simulink model "swing_language_control_sim"  (R2025a)
settings: Solver=ode4  StartTime=0.0  StopTime=simDuration  FixedStep=0.1  RelTol=1e-3
values from neighbouring files (symbols this model uses):
  siteMap = jsondecode(fileread(mapPath))    [actionsToVelocityCmd.m]
settings Model: Creator=Lenovo  LastModifiedBy=Lenovo

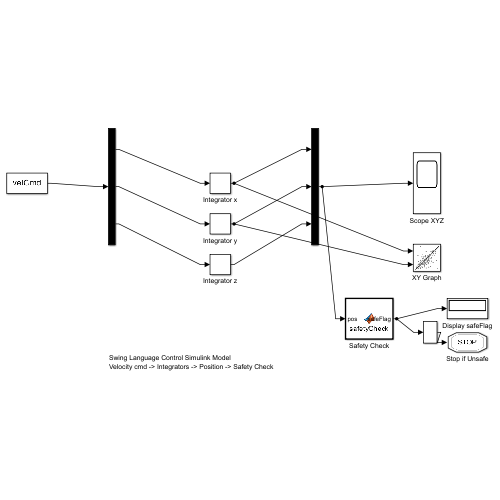
[thumbnail: Simulink's stored preview of the top-level diagram]
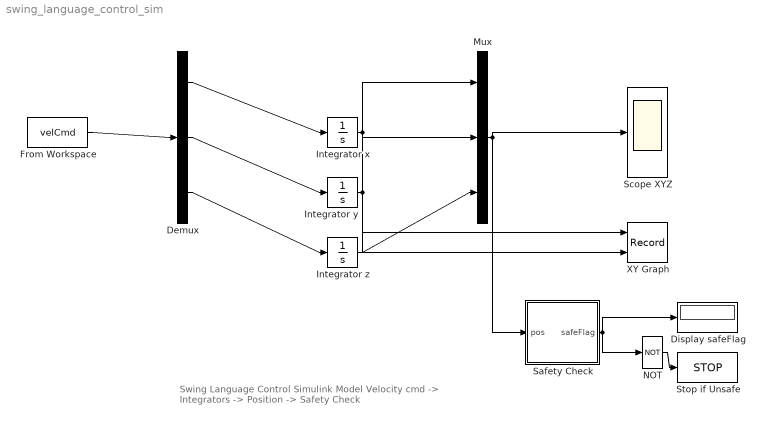
== system swing_language_control_sim ==
  note: Swing Language Control Simulink Model
      | Velocity cmd -> Integrators -> Position -> Safety Check
  Demux : Demux  Outputs=3
  Display safeFlag : Display
  From Workspace : FromWorkspace  VariableName=velCmd
  Integrator x : Integrator  InitialCondition=siteMap.origin.x
  Integrator y : Integrator  InitialCondition=siteMap.origin.y
  Integrator z : Integrator  InitialCondition=siteMap.origin.z
  Mux : Mux  Inputs=3
  NOT : Logic  Operator=NOT  AllPortsSameDT=off  OutDataTypeStr=boolean
  Safety Check : MATLAB Function  TreatAsAtomicUnit=on
  Scope XYZ : Scope
  Stop if Unsafe : Stop
  XY Graph : Record  NumPorts=2.0  FileSettingsInternal="{\"entries\":[{\"content\":{\"excelSettings\":{\"content\":{},\"type\":\"Streamout.ExcelSettings\"},\"parquetSettings\":{\"content\":{},\"type\":\"Streamout.ParquetSettings\"}},\"type\":\"Streamout.FileSettingStorage\",\"uuid\":\"\"}],\"packageUris\":[\"http:\\/\\/schema.mathworks.com\\/mf0\\/streamout_blocks\\/R2020a\"],\"version\":\"1.0\"}"  FrameSettings=[0, 0]  Layout=[1 1]  SignalsInternal="{\"entries\":[{\"content\":{\"signals\":[{\"content\":{\"blockPath\":[],\"dimensions\":[1],\"domain\":\"\",\"lineColor\":\"#a2142f\",\"plots\":[ 1 ],\"port\":1,\"sid\":[\"\"],\"signalID\":1,\"signalName\":\"Integrator x\"},\"type\":\"RecordBlkView.Signal\",\"uuid\":\"\"},{\"content\":{\"blockPath\":[],\"dimensions\":[1],\"domain\":\"\",\"lineColor\":\"#139fff\",\"plots\":[ 1 ],\"port\":2,\"sid\":[\"\"],\"signalID\":2,\"signalName\":\"Integrator y\"},\"type\":\"RecordBlkView.Signal\",\"uuid\":\"\"}]},\"type\":\"RecordBlkView.InputSignals\",\"uuid\":\"\"}],\"packageUris\":[\"http:\\/\\/schema.mathworks.com\\/mf0\\/streamout_blocks\\/R2020a\"],\"version\":\"1.0\"}"  VisualizationBindings="{\"xyplotplugin\":{\"info\":[{\"series\":[{\"bindingParametersList\":[{\"parameter\":\"X-Axis\",\"signalID\":1,\"signalName\":\"Integrator x\"},{\"parameter\":\"Y-Axis\",\"signalID\":2,\"signalName\":\"Integrator y\"}],\"seriesID\":0}],\"subplotID\":1}]}}"  CompatibilityTag=XY
  wires:
  From Workspace/1 -> Demux/1
  Demux/1 -> Integrator x/1
  Integrator x/1 -> Mux/1, XY Graph/1
  Demux/2 -> Integrator y/1
  Integrator y/1 -> Mux/2, XY Graph/2
  Demux/3 -> Integrator z/1
  Integrator z/1 -> Mux/3
  Mux/1 -> Scope XYZ/1, Safety Check/1(pos)
  Safety Check/1(safeFlag) -> Display safeFlag/1, NOT/1
  NOT/1 -> Stop if Unsafe/1

== matlab function swing_language_control_sim/Safety Check ==
  data: pos input; safeFlag output
function safeFlag = safetyCheck(pos)
%#codegen
safeFlag = 1;
x = pos(1); y = pos(2); z = pos(3);
limits = [-6 6 -6 6 0 3];
zones = [1.5 1.2 1.3;-1.5 0.80000000000000004 1];
if x < limits(1) || x > limits(2) || ...
        y < limits(3) || y > limits(4) || ...
        z < limits(5) || z > limits(6)
    safeFlag = 0; return;
end
for i = 1:size(zones, 1)
    dist = hypot(x - zones(i, 1), y - zones(i, 2));
    if dist <= zones(i, 3)
        safeFlag = 0; return;
    end
end
end
